simulink model "pendulum_control_linear"  (R2018b)
settings: Solver=VariableStepAuto  StartTime=0.0  StopTime=10.0  RelTol=1e-3
values from neighbouring files (symbols this model uses):
  A = [0 1 0 0;(g/L) 0 0 0; 0 0 0 1; 0 0 0 0]    [inverted_pendulum.m]    (also in inverted_pendulum_final.m)
  A_aug = [0 -C_bot; zeros(4,1) A]    [inverted_pendulum.m]    (also in inverted_pendulum_final.m)
  alpha = 0.5    [inverted_pendulum.m]    (also in inverted_pendulum_final.m = 0.9)
  B = [0; -(1/L); 0; 1]    [inverted_pendulum.m]    (also in inverted_pendulum_final.m)
  B_aug = [-D_bot; B]    [inverted_pendulum.m]    (also in inverted_pendulum_final.m)
  Br_aug = [1; zeros(4,1)]    [inverted_pendulum.m]    (also in inverted_pendulum_final.m)
  Bw_aug = B_aug    [inverted_pendulum.m]    (also in inverted_pendulum_final.m)
  C = [1 0 0 0; 0 0 1 0]    [inverted_pendulum.m]    (also in inverted_pendulum_final.m)
  C_aug = [C zeros(2,1)]    [inverted_pendulum.m]    (also in inverted_pendulum_final.m = [zeros(2,1) C])
  D = [0; 0]    [inverted_pendulum.m]    (also in inverted_pendulum_final.m)
  ICo = 0    [inverted_pendulum.m]    (also in inverted_pendulum_final.m)
  kbar = kpoles(2:end)    [inverted_pendulum.m]    (also in inverted_pendulum_final.m)
  ki = -kpoles(1)    [inverted_pendulum.m]    (also in inverted_pendulum_final.m = kpoles(1))
  lbar = place(A', C', pe)'    [inverted_pendulum.m]    (also in inverted_pendulum_final.m)
settings Model: Creator=ipebo  LastModifiedBy=ipebo
settings DataIOCC: SaveFormat=Structure

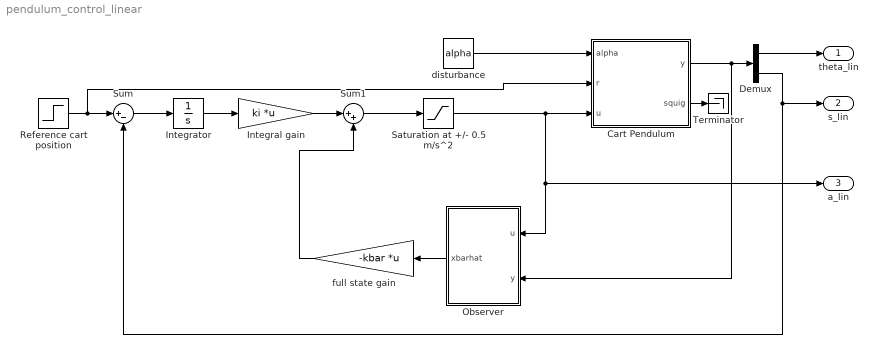
== system pendulum_control_linear ==
  Cart Pendulum : Subsystem
  Demux : Demux  Outputs=2
  Integral gain : Gain  Gain=ki  Multiplication=Matrix(K*u) (u vector)
  Integrator : Integrator
  Observer : Subsystem
  Reference cart position : Step  SampleTime=0
  Saturation at +/- 0.5 m/s^2 : Saturate
  Sum : Sum  Inputs=|+-
  Sum1 : Sum  Inputs=|++
  Terminator : Terminator
  disturbance : Constant  Value=alpha
  full state gain : Gain  Gain=-kbar  Multiplication=Matrix(K*u) (u vector)
  theta_lin : Outport  SignalName=theta_lin
  s_lin : Outport  Port=2  SignalName=s_lin
  a_lin : Outport  Port=3  SignalName=a_lin
  wires:
  Reference cart position/1 -> Cart Pendulum/2(r), Sum/1
  Sum/1 -> Integrator/1
  Integrator/1 -> Integral gain/1
  Integral gain/1 -> Sum1/1
  Sum1/1 -> Saturation at +/- 0.5 m/s^2/1
  full state gain/1 -> Sum1/2
  Saturation at +/- 0.5 m/s^2/1 -> Cart Pendulum/3(u), Observer/1(u), a_lin/1
  Observer/1(xbarhat) -> full state gain/1
  disturbance/1 -> Cart Pendulum/1(alpha)
  Demux/1 -> theta_lin/1
  Demux/2 -> s_lin/1, Sum/2
  Cart Pendulum/2(squig) -> Terminator/1
  Cart Pendulum/1(y) -> Demux/1, Observer/2(y)

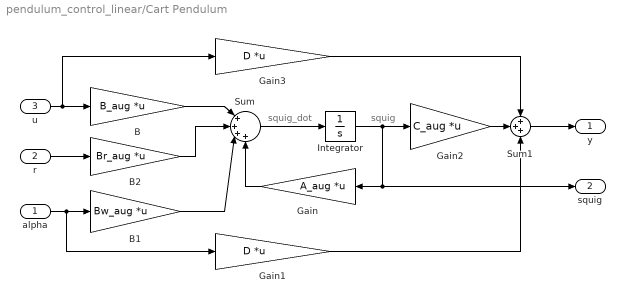
== system pendulum_control_linear/Cart Pendulum ==
  note: squig
  note: squig_dot
  alpha : Inport
  r : Inport  Port=2
  u : Inport  Port=3
  B : Gain  Gain=B_aug  Multiplication=Matrix(K*u) (u vector)
  B1 : Gain  Gain=Bw_aug  Multiplication=Matrix(K*u) (u vector)
  B2 : Gain  Gain=Br_aug  Multiplication=Matrix(K*u) (u vector)
  Gain : Gain  Gain=A_aug  Multiplication=Matrix(K*u) (u vector)
  Gain1 : Gain  Gain=D  Multiplication=Matrix(K*u) (u vector)
  Gain2 : Gain  Gain=C_aug  Multiplication=Matrix(K*u) (u vector)
  Gain3 : Gain  Gain=D  Multiplication=Matrix(K*u) (u vector)
  Integrator : Integrator
  Sum : Sum  Inputs=|++++
  Sum1 : Sum  Inputs=+++
  y : Outport
  squig : Outport  Port=2
  wires:
  Sum1/1 -> y/1
  B/1 -> Sum/1
  Gain3/1 -> Sum1/1
  Integrator/1 -> Gain/1, squig/1, Gain2/1
  Sum/1 -> Integrator/1
  u/1 -> B/1, Gain3/1
  alpha/1 -> Gain1/1, B1/1
  r/1 -> B2/1
  Gain/1 -> Sum/4
  B2/1 -> Sum/2
  B1/1 -> Sum/3
  Gain1/1 -> Sum1/3
  Gain2/1 -> Sum1/2

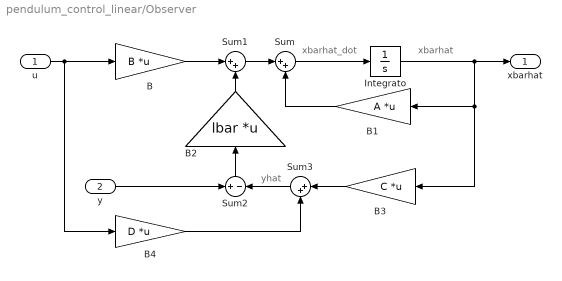
== system pendulum_control_linear/Observer ==
  note: xbarhat_dot
  note: xbarhat
  note: yhat
  u : Inport
  y : Inport  Port=2
  B : Gain  Gain=B  Multiplication=Matrix(K*u) (u vector)
  B1 : Gain  Gain=A  Multiplication=Matrix(K*u) (u vector)
  B2 : Gain  Gain=lbar  Multiplication=Matrix(K*u) (u vector)
  B3 : Gain  Gain=C  Multiplication=Matrix(K*u) (u vector)
  B4 : Gain  Gain=D  Multiplication=Matrix(K*u) (u vector)
  Integrato : Integrator  InitialCondition=ICo
  Sum : Sum  Inputs=|++
  Sum1 : Sum  Inputs=|++
  Sum2 : Sum  Inputs=+-
  Sum3 : Sum  Inputs=|++
  xbarhat : Outport
  wires:
  u/1 -> B/1, B4/1
  B4/1 -> Sum3/2
  y/1 -> Sum2/1
  B/1 -> Sum1/1
  Sum3/1 -> Sum2/2
  Integrato/1 -> xbarhat/1, B1/1, B3/1
  B3/1 -> Sum3/1
  Sum1/1 -> Sum/1
  B2/1 -> Sum1/2
  B1/1 -> Sum/2
  Sum/1 -> Integrato/1
  Sum2/1 -> B2/1
